simulink model "System_Test"  (R2022b)
settings: Solver=FixedStepAuto  StartTime=0.0  StopTime=40  RelTol=1e-3  EnableMultiTasking=on
undefined symbols (not defined in the file or in its folder): Ri, Rw, sat, uc
libraries: arduinolib x4, simulink x2, eeGeneralControl x1, dspfdesign x1, dspsigops x1
settings Model: SimulationMode=external  ExtModeTrigDuration=2  Creator=gotta  LastModifiedBy=gotta
settings OptimizationCC: EnhancedBackFolding=on  PassReuseOutputArgsAs=Individual arguments  ZeroExternalMemoryAtStartup=off  ZeroInternalMemoryAtStartup=off  MaxStackSize=64  OptimizeBlockOrder=speed  DifferentSizesBufferReuse=on  OptimizationCustomize=off  EfficientTunableParamExpr=on
settings DebuggingCC: ParameterTunabilityLossMsg=error
settings HardwareCC: ProdBitPerPointer=32  ProdBitPerSizeT=32  ProdBitPerPtrDiffT=32  ProdLargestAtomicInteger=Long  ProdLargestAtomicFloat=Double  ProdWordSize=32  ProdHWDeviceType=ARM Compatible->ARM Cortex
settings SFSimCC: MATLABDynamicMemAlloc=off
settings RTWCC: Description=Embedded Coder  SystemTargetFile=ert.tlc  HardwareBoard=ESP32-WROOM(Arduino Compatible)  TLCOptions="-aInlineSetEventsForThisBaseRateFcn=TLC_FALSE -aSuppressMultiTaskScheduler=TLC_FALSE  -aRateBasedStepFcn=0"  TemplateMakefile=ert_default_tmf  Toolchain=ESP32  BuildConfiguration=Faster Runs
settings CodeAppCC: ForceParamTrailComments=on  IgnoreCustomStorageClasses=off  OperatorAnnotations=on  SimulinkDataObjDesc=on  SFDataObjDesc=on  InsertBlockDesc=on
settings ERTTargetCC: SupportContinuousTime=on  SupportVariableSizeSignals=on  ExtModeTransport=3  ExtModeStaticAlloc=on  ExtModeAutomaticAllocSize=off  ExtModeStaticAllocSize=65536  ExtModeMexFile=ext_xcp  ExtModeIntrfLevel=Level2 - Open

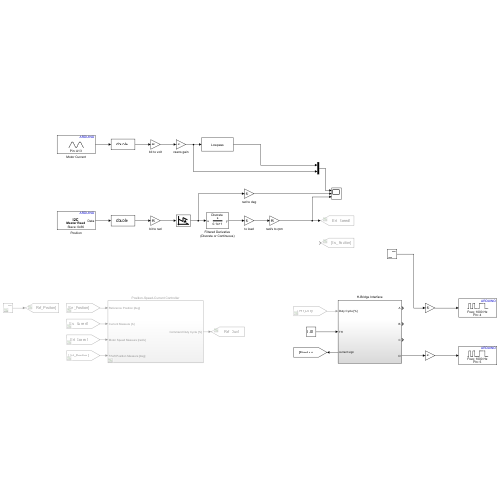
[thumbnail: Simulink's stored preview of the top-level diagram]
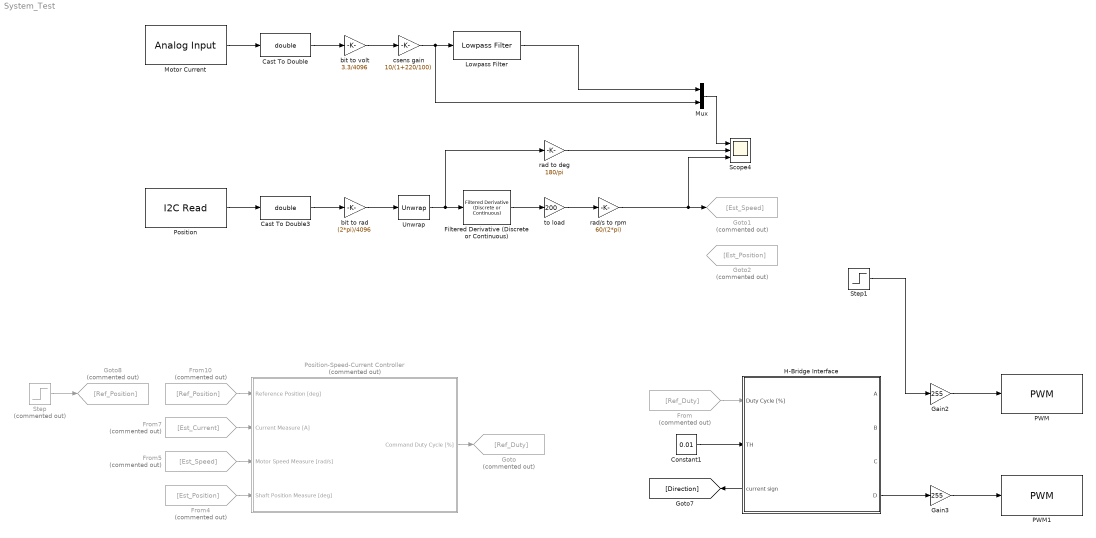
== system System_Test ==
  Cast To Double : DataTypeConversion  OutDataTypeStr=double  SaturateOnIntegerOverflow=off  RndMeth=Floor
  Cast To Double3 : DataTypeConversion  OutDataTypeStr=double  SaturateOnIntegerOverflow=off  RndMeth=Floor
  Constant1 : Constant  Value=0.01
  Filtered Derivative (Discrete or Continuous) : eeGeneralControl/Filtered Derivative (Discrete or Continuous)  K=1  T=0.1  B=inf  A=-inf  minRatio=10  init_option=Inherited from block input  x0=0  Ts=0.001
      settings: LibrarySourceBlock=|
      | ee_sl_lib/General Control/Filtered Derivative
      | (Discrete or Continuous)
  From : From  Commented=on  GotoTag=Ref_Duty
  From10 : From  Commented=on  GotoTag=Ref_Position
  From4 : From  Commented=on  GotoTag=Est_Position
  From5 : From  Commented=on  GotoTag=Est_Speed
  From7 : From  Commented=on  GotoTag=Est_Current
  Gain2 : Gain  Gain=255
  Gain3 : Gain  Gain=255
  Goto : Goto  Commented=on  GotoTag=Ref_Duty
  Goto1 : Goto  Commented=on  GotoTag=Est_Speed
  Goto2 : Goto  Commented=on  GotoTag=Est_Position
  Goto8 : Goto  Commented=on  GotoTag=Ref_Position
  H-Bridge Interface : Subsystem
      settings: PortSchema="{\"entries\":[{\"content\":{\"sides\":[{\"content\":{\"connectorIds\":[\"In1\",\"In2\",\"Out5\"]},\"type\":\"ConnectorPlacement.EquallySpacedRectSide\",\"uuid\":\"3e1f6d45-7616-4063-a130-e4013823fbd2\"},{\"content\":{\"connectorIds\":[\"Out1\",\"Out2\",\"Out3\",\"Out4\"],\"side\":\"RIGHT\"},\"type\":\"ConnectorPlacement.EquallySpacedRectSide\",\"uuid\":\"9e6093c0-e90e-442b-85bd-caf841044685\"},{\"content\":{\"connectorIds\":[],\"side\":\"TOP\"},\"type\":\"ConnectorPlacement.EquallySpacedRectSide\",\"uuid\":\"c5091c1c-d592-4b25-a882-dfd9d3329f63\"}]},\"type\":\"ConnectorPlacement.EquallySpacedConnector\",\"uuid\":\"99d9d6e0-cfe7-4913-a6cd-9e1192c47eae\"}],\"packageUris\":[\"http://schema.mathworks.com/mf0/Connector/R2020b\"],\"version\":\"1.0\"}"
  Lowpass Filter : dspfdesign/Lowpass Filter  FilterType=FIR  DesignForMinimumOrder=on  FilterOrder=50  PassbandFrequency=4000  StopbandFrequency=5000  PassbandRipple=0.1  StopbandAttenuation=80  InheritSampleRate=off  SampleRate=44100  SimulateUsing=Interpreted execution  roundingMode=Floor  coeffsDataTypeStr=fixdt(1,16)
  Motor Current : arduinolib/Analog Input  pinNumber=13  ReadResultsOnly=off  ConversionTriggerSource=Software  ExternalTriggerType=uint32( 0 )  OutputDataType=uint16  EnableConversionCompleteNotify=off  EnableOuputStatus=off  SampleTime=0.001  blockPlatform=arduino
  Mux : Mux  Inputs=2
  PWM : arduinolib/PWM  pinNumber=4  frequencyType=Specify  desiredFrequency=1000  achievableFrequency=1000
  PWM1 : arduinolib/PWM  pinNumber=5  frequencyType=Specify  desiredFrequency=1000  achievableFrequency=1000
  Position : arduinolib/I2C Read  I2CModule=0  Mode=Master  SlaveAddress=0x36  SlaveByteOrder=BigEndian  Direction=Receiver  RegisterAddressMode=on  RegisterAddress=0x0E  SlaveDataType=int16  DataLength=1  NoAck=off  RepeatedStart=off  OutputStatus=off  blockPlatform=ARDUINO  SampleTime=uc.Ts
  Position-Speed-Current Controller : Subsystem  Commented=on
  Scope4 : Scope  NumInputPorts=3
  Step : Step  Commented=on  Time=0.1  After=170  SampleTime=uc.Ts
  Step1 : Step  SampleTime=0
  Unwrap : dspsigops/Unwrap  tol=pi  InputProcessing=Columns as channels (frame based)  running=off
  bit to rad : Gain  Gain=(2*pi)/4096
  bit to volt : Gain  Gain=3.3/4096
  csens gain : Gain  Gain=10/(1+220/100)
  rad to deg : Gain  Gain=180/pi
  rad/s to rpm : Gain  Gain=60/(2*pi)
  to load : Gain  Gain=200
  wires:
  Motor Current/1 -> Cast To Double/1
  Cast To Double/1 -> bit to volt/1
  Position/1 -> Cast To Double3/1
  Cast To Double3/1 -> bit to rad/1
  Position-Speed-Current Controller/1(Command Duty Cycle [%]) -> Goto/1
  From10/1 -> Position-Speed-Current Controller/1(Reference Position [deg])
  Step/1 -> Goto8/1
  H-Bridge Interface/5(current sign) -> [Direction]
  From7/1 -> Position-Speed-Current Controller/2(Current Measure [A])
  From5/1 -> Position-Speed-Current Controller/3(Motor Speed Measure [rad/s])
  Constant1/1 -> H-Bridge Interface/2(TH)
  From4/1 -> Position-Speed-Current Controller/4(Shaft Position Measure [deg])
  Filtered Derivative (Discrete or Continuous)/1 -> to load/1
  to load/1 -> rad/s to rpm/1
  rad/s to rpm/1 -> Goto1/1, Scope4/3
  bit to volt/1 -> csens gain/1
  csens gain/1 -> Mux/2, Lowpass Filter/1
  Gain2/1 -> PWM/1
  Gain3/1 -> PWM1/1
  bit to rad/1 -> Unwrap/1
  Unwrap/1 -> Filtered Derivative (Discrete or Continuous)/1, rad to deg/1
  rad to deg/1 -> Scope4/2
  Lowpass Filter/1 -> Mux/1
  Mux/1 -> Scope4/1
  H-Bridge Interface/4(D) -> Gain3/1
  From/1 -> H-Bridge Interface/1(Duty Cycle [%])
  Step1/1 -> Gain2/1

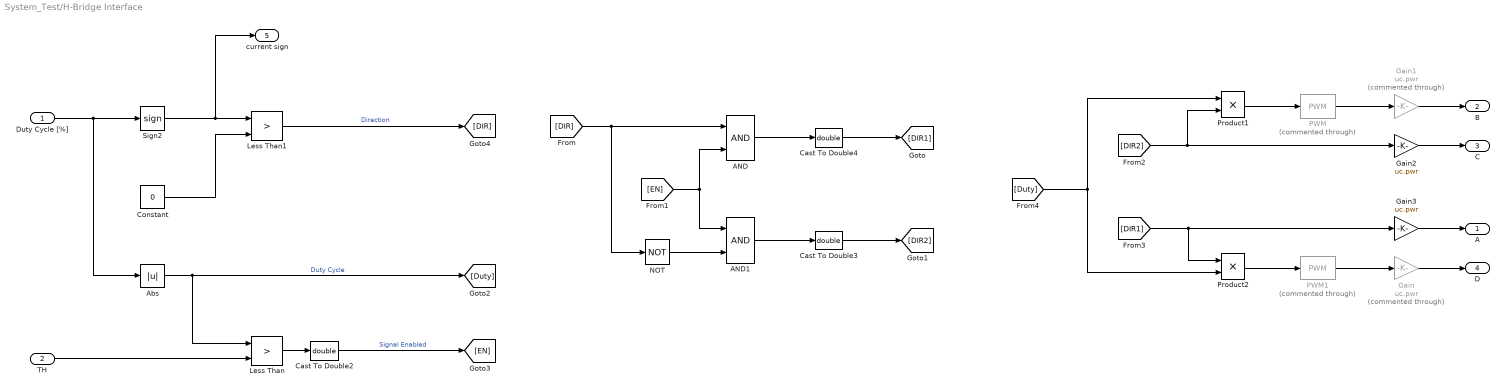
== system System_Test/H-Bridge Interface ==
  Duty Cycle [%] : Inport
  TH : Inport  Port=2
  AND : Logic  IconShape=distinctive  AllPortsSameDT=off  OutDataTypeStr=boolean
  AND1 : Logic  IconShape=distinctive  AllPortsSameDT=off  OutDataTypeStr=boolean
  Abs : Abs  SaturateOnIntegerOverflow=off
  Cast To Double2 : DataTypeConversion  OutDataTypeStr=double  SaturateOnIntegerOverflow=off  RndMeth=Floor
  Cast To Double3 : DataTypeConversion  OutDataTypeStr=double  SaturateOnIntegerOverflow=off  RndMeth=Floor
  Cast To Double4 : DataTypeConversion  OutDataTypeStr=double  SaturateOnIntegerOverflow=off  RndMeth=Floor
  Constant : Constant  Value=0
  Gain : Gain  Commented=through  Gain=uc.pwr
  Gain1 : Gain  Commented=through  Gain=uc.pwr
  Gain2 : Gain  Gain=uc.pwr
  Gain3 : Gain  Gain=uc.pwr
  Less Than : RelationalOperator  Operator=>  OutDataTypeStr=boolean  RndMeth=Simplest  InputSameDT=off
  Less Than1 : RelationalOperator  Operator=>  OutDataTypeStr=boolean  RndMeth=Simplest  InputSameDT=off
  NOT : Logic  Operator=NOT  IconShape=distinctive  AllPortsSameDT=off  OutDataTypeStr=boolean
  PWM : simulink/Discontinuities/PWM  Commented=through  DisableCoverage=on  Period=uc.Tpwm  InitialDelay=0  DisallowZeroDutyCycle=off  RunAtFixedTimeIntervals=on  SampleTime=uc.Tpwm/10
  PWM1 : simulink/Discontinuities/PWM  Commented=through  DisableCoverage=on  Period=uc.Tpwm  InitialDelay=0  DisallowZeroDutyCycle=off  RunAtFixedTimeIntervals=on  SampleTime=uc.Tpwm/10
  Product1 : Product
  Product2 : Product
  Sign2 : Signum
  A : Outport
  B : Outport  Port=2
  C : Outport  Port=3
  D : Outport  Port=4
  current sign : Outport  Port=5
  wires:
  TH/1 -> Less Than/2
  Duty Cycle [%]/1 -> Abs/1, Sign2/1
  Less Than/1 -> Cast To Double2/1
  Sign2/1 -> current sign/1, Less Than1/1
  Constant/1 -> Less Than1/2
  Abs/1 -> [Duty], Less Than/1  "Duty Cycle"
  Gain/1 -> D/1
  Gain1/1 -> B/1
  Gain2/1 -> C/1
  Gain3/1 -> A/1
  AND1/1 -> Cast To Double3/1
  AND/1 -> Cast To Double4/1
  NOT/1 -> AND1/2
  Product1/1 -> PWM/1
  Product2/1 -> PWM1/1
  Cast To Double2/1 -> [EN]  "Signal Enabled"
  Less Than1/1 -> [DIR]  "Direction"
  [DIR] -> NOT/1, AND/1
  [EN] -> AND/2, AND1/1
  Cast To Double4/1 -> [DIR1]
  Cast To Double3/1 -> [DIR2]
  [DIR2] -> Product1/2, Gain2/1
  [DIR1] -> Product2/1, Gain3/1
  [Duty] -> Product1/1, Product2/2
  PWM/1 -> Gain1/1
  PWM1/1 -> Gain/1

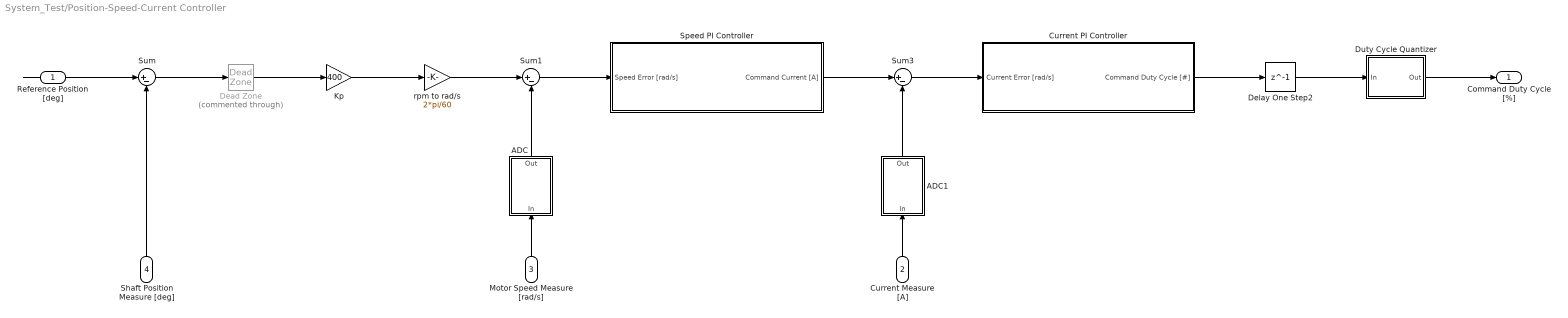
== system System_Test/Position-Speed-Current Controller ==
  Reference Position [deg] : Inport
  Current Measure [A] : Inport  Port=2
  Motor Speed Measure [rad/s] : Inport  Port=3
  Shaft Position Measure [deg] : Inport  Port=4
  ADC : Subsystem
  ADC1 : Subsystem
  Current PI Controller : Subsystem
  Dead Zone : DeadZone  Commented=through
  Delay One Step2 : Delay  DelayLength=1
  Duty Cycle Quantizer : Subsystem
  Kp : Gain  Gain=400
  Speed PI Controller : Subsystem
  Sum : Sum  Inputs=|+-
  Sum1 : Sum  Inputs=|+-
  Sum3 : Sum  Inputs=|+-
  rpm to rad/s : Gain  Gain=2*pi/60
  Command Duty Cycle [%] : Outport
  wires:
  Kp/1 -> rpm to rad/s/1
  Speed PI Controller/1(Command Current [A]) -> Sum3/1
  Current PI Controller/1(Command Duty Cycle [#]) -> Delay One Step2/1
  rpm to rad/s/1 -> Sum1/1
  Sum/1 -> Dead Zone/1
  Sum3/1 -> Current PI Controller/1(Current Error [rad/s])
  Reference Position [deg]/1 -> Sum/1
  Sum1/1 -> Speed PI Controller/1(Speed Error [rad/s])
  Current Measure [A]/1 -> ADC1/1(In)
  Shaft Position Measure [deg]/1 -> Sum/2
  Motor Speed Measure [rad/s]/1 -> ADC/1(In)
  Delay One Step2/1 -> Duty Cycle Quantizer/1(In)
  Duty Cycle Quantizer/1(Out) -> Command Duty Cycle [%]/1
  ADC1/1(Out) -> Sum3/2
  ADC/1(Out) -> Sum1/2
  Dead Zone/1 -> Kp/1

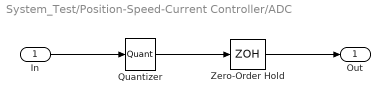
== system System_Test/Position-Speed-Current Controller/ADC ==
  In : Inport
  Quantizer : Quantizer  QuantizationInterval=uc.adc_q
  Zero-Order Hold : ZeroOrderHold  SampleTime=uc.Ts
  Out : Outport
  wires:
  Quantizer/1 -> Zero-Order Hold/1
  Zero-Order Hold/1 -> Out/1
  In/1 -> Quantizer/1

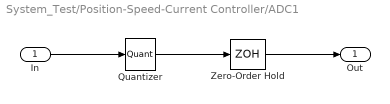
== system System_Test/Position-Speed-Current Controller/ADC1 ==
  In : Inport
  Quantizer : Quantizer  QuantizationInterval=uc.adc_q
  Zero-Order Hold : ZeroOrderHold  SampleTime=uc.Ts
  Out : Outport
  wires:
  Quantizer/1 -> Zero-Order Hold/1
  Zero-Order Hold/1 -> Out/1
  In/1 -> Quantizer/1

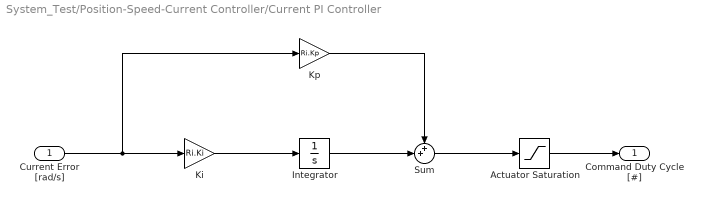
== system System_Test/Position-Speed-Current Controller/Current PI Controller ==
  Current Error [rad/s] : Inport
  Actuator Saturation : Saturate  UpperLimit=sat.d  LowerLimit=-sat.d
  Integrator : Integrator  LimitOutput=on  UpperSaturationLimit=sat.d  LowerSaturationLimit=-sat.d
  Ki : Gain  Gain=Ri.Ki
  Kp : Gain  Gain=Ri.Kp
  Sum : Sum  Inputs=++|
  Command Duty Cycle [#] : Outport
  wires:
  Integrator/1 -> Sum/2
  Ki/1 -> Integrator/1
  Sum/1 -> Actuator Saturation/1
  Kp/1 -> Sum/1
  Current Error [rad/s]/1 -> Ki/1, Kp/1
  Actuator Saturation/1 -> Command Duty Cycle [#]/1

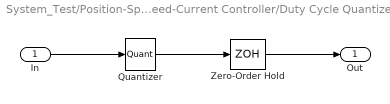
== system System_Test/Position-Speed-Current Controller/Duty Cycle Quantizer ==
  In : Inport
  Quantizer : Quantizer  QuantizationInterval=uc.duty_step
  Zero-Order Hold : ZeroOrderHold  SampleTime=uc.Ts
  Out : Outport
  wires:
  Quantizer/1 -> Zero-Order Hold/1
  Zero-Order Hold/1 -> Out/1
  In/1 -> Quantizer/1

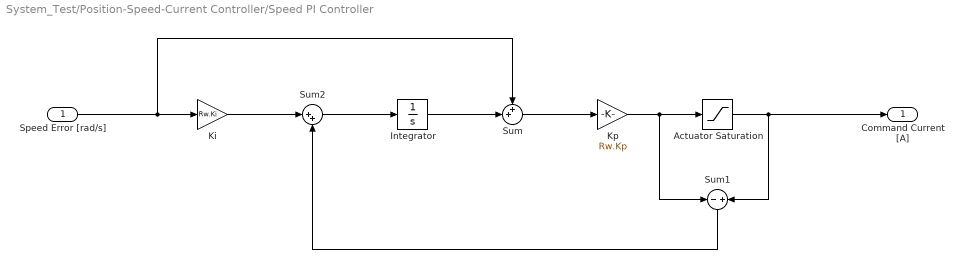
== system System_Test/Position-Speed-Current Controller/Speed PI Controller ==
  Speed Error [rad/s] : Inport
  Actuator Saturation : Saturate  UpperLimit=sat.I  LowerLimit=-sat.I
  Integrator : Integrator  LimitOutput=on  UpperSaturationLimit=sat.I  LowerSaturationLimit=-sat.I
  Ki : Gain  Gain=Rw.Ki
  Kp : Gain  Gain=Rw.Kp
  Sum : Sum  Inputs=++|
  Sum1 : Sum  Inputs=-+
  Sum2 : Sum  Inputs=|++
  Command Current [A] : Outport
  wires:
  Integrator/1 -> Sum/2
  Sum/1 -> Kp/1
  Ki/1 -> Sum2/1
  Sum2/1 -> Integrator/1
  Sum1/1 -> Sum2/2
  Kp/1 -> Actuator Saturation/1, Sum1/1
  Speed Error [rad/s]/1 -> Sum/1, Ki/1
  Actuator Saturation/1 -> Command Current [A]/1, Sum1/2
